simulink model "FIR_filter"  (R2020b)
settings: Solver=FixedStepAuto  StartTime=0.0  StopTime=10.0  FixedStep=0.2  RelTol=1e-3
settings Model: Creator=DELL  LastModifiedBy=DELL
settings DataIOCC: SaveOutput=off  SaveTime=off

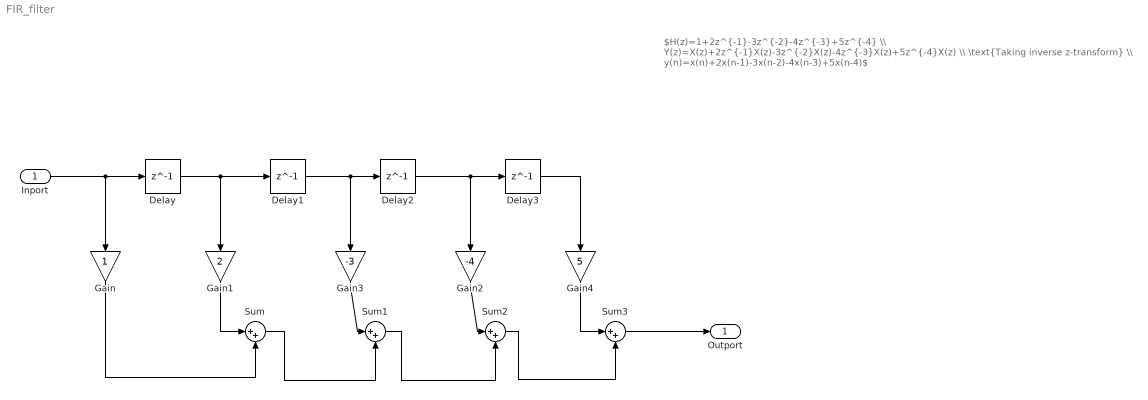
== system FIR_filter ==
  note: $H(z)=1+2z^{-1}-3z^{-2}-4z^{-3}+5z^{-4} \\ Y(z)=X(z)+2z^{-1}X(z)-3z^{-2}X(z)-4z^{-3}X(z)+5z^{-4}X(z) \\ \text{Taking inverse z-transform} \\ y(n)=x(n)+2x(n-1)-3x(n-2)-4x(n-3)+5x(n-4)$
  Inport : Inport  OutDataTypeStr=double  PortDimensions=1  SampleTime=[0.20000000000000001,0]
  Delay{,1..3} (4 alike) : Delay  DelayLength=1
  Gain : Gain
  Gain1 : Gain  Gain=2
  Gain2 : Gain  Gain=-4
  Gain3 : Gain  Gain=-3
  Gain4 : Gain  Gain=5
  Sum{,1..3} (4 alike) : Sum  Inputs=|++
  Outport : Outport  OutDataTypeStr=double  PortDimensions=1  SampleTime=[0.20000000000000001,0]
  wires:
  Delay3/1 -> Gain4/1
  Gain3/1 -> Sum1/1
  Sum3/1 -> Outport/1
  Delay2/1 -> Delay3/1, Gain2/1
  Inport/1 -> Delay/1, Gain/1
  Sum2/1 -> Sum3/2
  Delay/1 -> Delay1/1, Gain1/1
  Gain/1 -> Sum/2
  Delay1/1 -> Delay2/1, Gain3/1
  Sum1/1 -> Sum2/2
  Gain1/1 -> Sum/1
  Sum/1 -> Sum1/2
  Gain2/1 -> Sum2/1
  Gain4/1 -> Sum3/1
